simulink model "NlinCloopQuadrotor"  (R2021a)
settings: Solver=VariableStepAuto  StartTime=0.0  StopTime=100.0  RelTol=1e-3
values from neighbouring files (symbols this model uses):
  g = 9.8    [Linearmodel.m]
  J = diag([2.7,3.3,5.4])    [Linearmodel.m]
  Jinv = J^-1    [Linearmodel.m]
  m = 0.254    [Linearmodel.m]
settings Model: Creator=Sirius  LastModifiedBy=Sirius

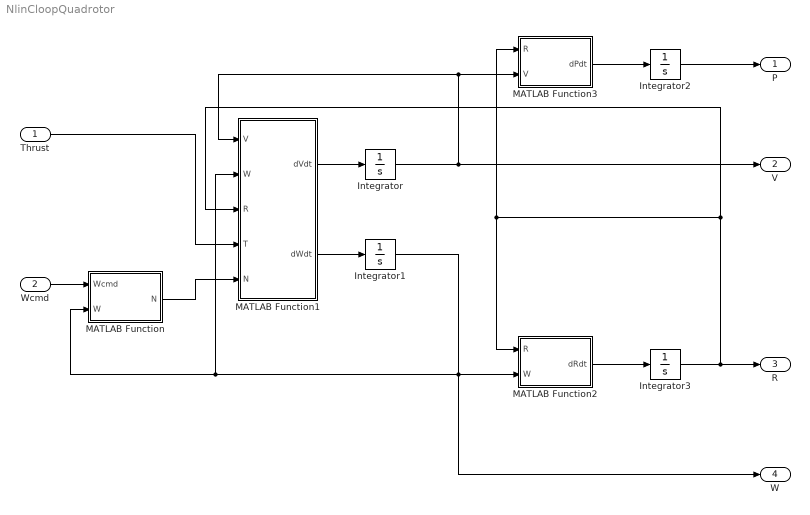
== system NlinCloopQuadrotor ==
  Thrust : Inport
  Wcmd : Inport  Port=2
  Integrator : Integrator  InitialCondition=[0;0;0]
  Integrator1 : Integrator  InitialCondition=[0;0;0]
  Integrator2 : Integrator  InitialCondition=[0;1;0]
  Integrator3 : Integrator  InitialCondition=eye(3)
  MATLAB Function : MATLAB Function  TreatAsAtomicUnit=on
  MATLAB Function1 : MATLAB Function  TreatAsAtomicUnit=on
  MATLAB Function2 : MATLAB Function  TreatAsAtomicUnit=on
  MATLAB Function3 : MATLAB Function  TreatAsAtomicUnit=on
  P : Outport
  V : Outport  Port=2
  R : Outport  Port=3
  W : Outport  Port=4
  wires:
  Thrust/1 -> MATLAB Function1/4(T)
  Wcmd/1 -> MATLAB Function/1(Wcmd)
  MATLAB Function1/1(dVdt) -> Integrator/1
  MATLAB Function1/2(dWdt) -> Integrator1/1
  MATLAB Function3/1(dPdt) -> Integrator2/1
  MATLAB Function2/1(dRdt) -> Integrator3/1
  Integrator/1 -> V/1, MATLAB Function1/1(V), MATLAB Function3/2(V)
  Integrator1/1 -> MATLAB Function1/2(W), MATLAB Function/2(W), W/1, MATLAB Function2/2(W)
  Integrator3/1 -> MATLAB Function1/3(R), MATLAB Function3/1(R), MATLAB Function2/1(R), R/1
  Integrator2/1 -> P/1
  MATLAB Function/1(N) -> MATLAB Function1/5(N)

== matlab function NlinCloopQuadrotor/MATLAB Function1 ==
  data: V input; dVdt output; W input; R input; T input; N input; dWdt output; Jinv parameter; m parameter; g parameter; J parameter
function [dVdt,dWdt]=QDyanamics(V,W,R,T,N,Jinv, m, g, J)
dVdt=-Skew(W)*V+1/m*([0;0;-T]+R'*[0;0;m*g]);
dWdt=Jinv*Skew(W)*J*W+Jinv*N;
end

== matlab function NlinCloopQuadrotor/MATLAB Function ==
  data: Wcmd input; N output; W input
function N = Wcontorl(Wcmd,W)
N=1000*(Wcmd-W);
end

== matlab function NlinCloopQuadrotor/MATLAB Function2 ==
  data: R input; dRdt output; W input
function dRdt=dRdt(R,W)
dRdt=R*Skew(W);
end

== matlab function NlinCloopQuadrotor/MATLAB Function3 ==
  data: R input; dPdt output; V input
function dPdt=dPdt(R,V)
dPdt=R*V;
end
